simulink model "PID_motor"  (R2019b)
settings: Solver=VariableStepAuto  StartTime=0.0  StopTime=30  RelTol=1e-3
PreLoadFcn:
  | load('turstin.m')
values from neighbouring files (symbols this model uses):
  b = 6.797e-04    (= 0.0006797)    [turstin.m]
  J = 0.007    [turstin.m]
  ke = 0.2154    [turstin.m]
  kt = 0.1186    [turstin.m]
  L = 0    [turstin.m]
  Nf = 100    [turstin.m]
  R = 2.400    (= 2.4)    [turstin.m]
  Tsample = 0.5    [turstin.m]
settings Model: Creator=Ommie  LastModifiedBy=Ommie

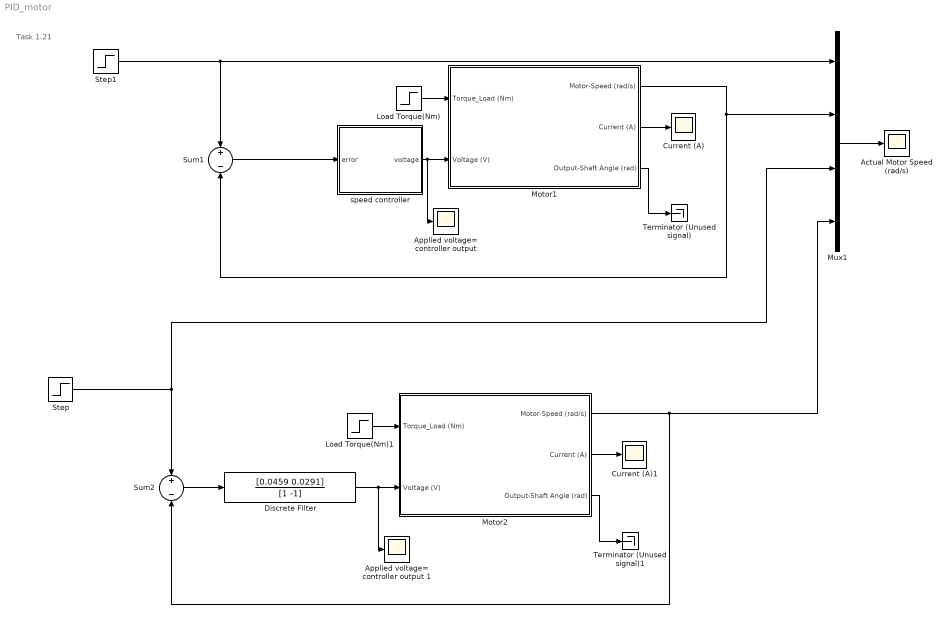
== system PID_motor ==
  note: Task 1.21
  Actual Motor Speed (rad/s) : Scope
  "Applied voltage= controller output " : Scope
  Applied voltage= controller output 1 : Scope
  Current (A) : Scope
  Current (A)1 : Scope
  "Discrete Filter " : DiscreteFilter  Numerator=[0.0459 0.0291]  Denominator=[1 -1]  SampleTime=Tsample
  Load Torque(Nm) : Step  Time=15  After=0.25  SampleTime=0
  Load Torque(Nm)1 : Step  Time=15  After=0.25  SampleTime=0
  Motor1 : Subsystem
  Motor2 : Subsystem
  Mux1 : Mux
  Step : Step  After=31.4  SampleTime=0
  Step1 : Step  After=31.4  SampleTime=0
  Sum1 : Sum  Inputs=+|-
  Sum2 : Sum  Inputs=+|-
  Terminator (Unused signal) : Terminator
  Terminator (Unused signal)1 : Terminator
  speed controller : Subsystem
  wires:
  speed controller/1(voltage) -> "Applied voltage= controller output "/1, Motor1/2(Voltage (V))
  Motor1/1(Motor-Speed (rad/s)) -> Sum1/2, Mux1/2
  Step1/1 -> Mux1/1, Sum1/1
  Mux1/1 -> Actual Motor Speed (rad/s)/1
  Motor1/3(Output-Shaft Angle (rad)) -> Terminator (Unused signal)/1
  Load Torque(Nm)/1 -> Motor1/1(Torque_Load (Nm))
  Sum1/1 -> speed controller/1(error)
  Motor1/2(Current (A)) -> Current (A)/1
  Step/1 -> Mux1/3, Sum2/1
  Motor2/2(Current (A)) -> Current (A)1/1
  "Discrete Filter "/1 -> Applied voltage= controller output 1/1, Motor2/2(Voltage (V))
  Load Torque(Nm)1/1 -> Motor2/1(Torque_Load (Nm))
  Sum2/1 -> "Discrete Filter "/1
  Motor2/3(Output-Shaft Angle (rad)) -> Terminator (Unused signal)1/1
  Motor2/1(Motor-Speed (rad/s)) -> Mux1/4, Sum2/2

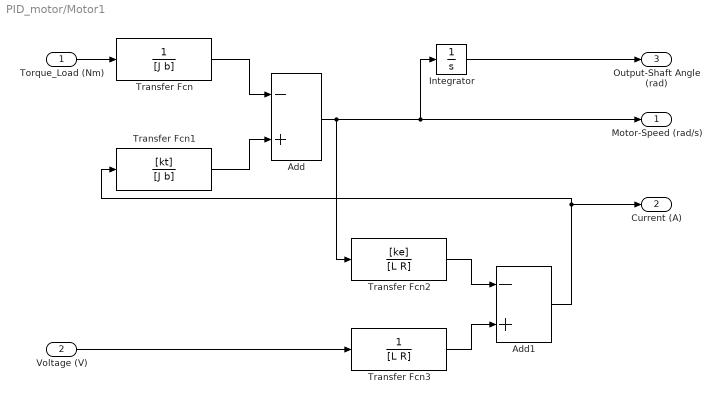
== system PID_motor/Motor1 ==
  Torque_Load (Nm) : Inport
  Voltage (V) : Inport  Port=2
  Add : Sum  Inputs=-+
  Add1 : Sum  Inputs=-+
  Integrator : Integrator
  Transfer Fcn : TransferFcn  Denominator=[J b]
  Transfer Fcn1 : TransferFcn  Numerator=[kt]  Denominator=[J b]
  Transfer Fcn2 : TransferFcn  Numerator=[ke]  Denominator=[L R]
  Transfer Fcn3 : TransferFcn  Numerator=1  Denominator=[L R]
  Motor-Speed (rad/s) : Outport  VectorParamsAs1DForOutWhenUnconnected=off
  Current (A) : Outport  Port=2  VectorParamsAs1DForOutWhenUnconnected=off
  Output-Shaft Angle (rad) : Outport  Port=3  VectorParamsAs1DForOutWhenUnconnected=off
  wires:
  Add1/1 -> Current (A)/1, Transfer Fcn1/1
  Torque_Load (Nm)/1 -> Transfer Fcn/1
  Transfer Fcn1/1 -> Add/2
  Integrator/1 -> Output-Shaft Angle (rad)/1
  Voltage (V)/1 -> Transfer Fcn3/1
  Transfer Fcn/1 -> Add/1
  Transfer Fcn2/1 -> Add1/1
  Transfer Fcn3/1 -> Add1/2
  Add/1 -> Motor-Speed (rad/s)/1, Integrator/1, Transfer Fcn2/1

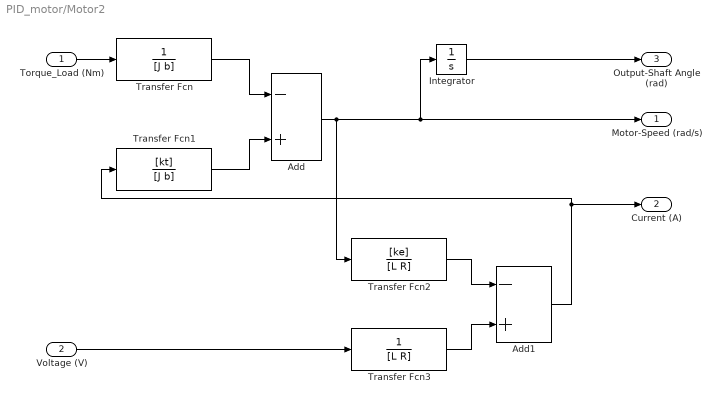
== system PID_motor/Motor2 ==
  Torque_Load (Nm) : Inport
  Voltage (V) : Inport  Port=2
  Add : Sum  Inputs=-+
  Add1 : Sum  Inputs=-+
  Integrator : Integrator
  Transfer Fcn : TransferFcn  Denominator=[J b]
  Transfer Fcn1 : TransferFcn  Numerator=[kt]  Denominator=[J b]
  Transfer Fcn2 : TransferFcn  Numerator=[ke]  Denominator=[L R]
  Transfer Fcn3 : TransferFcn  Numerator=1  Denominator=[L R]
  Motor-Speed (rad/s) : Outport  VectorParamsAs1DForOutWhenUnconnected=off
  Current (A) : Outport  Port=2  VectorParamsAs1DForOutWhenUnconnected=off
  Output-Shaft Angle (rad) : Outport  Port=3  VectorParamsAs1DForOutWhenUnconnected=off
  wires:
  Add1/1 -> Current (A)/1, Transfer Fcn1/1
  Torque_Load (Nm)/1 -> Transfer Fcn/1
  Transfer Fcn1/1 -> Add/2
  Integrator/1 -> Output-Shaft Angle (rad)/1
  Voltage (V)/1 -> Transfer Fcn3/1
  Transfer Fcn/1 -> Add/1
  Transfer Fcn2/1 -> Add1/1
  Transfer Fcn3/1 -> Add1/2
  Add/1 -> Motor-Speed (rad/s)/1, Integrator/1, Transfer Fcn2/1

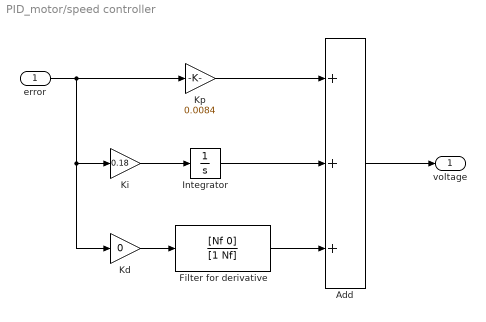
== system PID_motor/speed controller ==
  error : Inport
  Add : Sum  Inputs=+++
  Filter for derivative : TransferFcn  Numerator=[Nf 0]  Denominator=[1 Nf]
  Integrator : Integrator
  Kd : Gain  Gain=0
  Ki : Gain  Gain=0.18
  Kp : Gain  Gain=0.0084
  voltage : Outport  VectorParamsAs1DForOutWhenUnconnected=off
  wires:
  Filter for derivative/1 -> Add/3
  Kp/1 -> Add/1
  Integrator/1 -> Add/2
  error/1 -> Kd/1, Ki/1, Kp/1
  Add/1 -> voltage/1
  Ki/1 -> Integrator/1
  Kd/1 -> Filter for derivative/1
